simulink model "WESDem_SelectParam"  (R2016b)
settings: configuration reference "CodeGenConfigSet" (kept outside this file)
values from neighbouring files (symbols this model uses):
  WESDem_facFdbkHi_CUR = Calibration.Parameter    [init_WESDem_SelectParam.m]
  WESDem_facFdbkHi_CURX = Calibration.Parameter    [init_WESDem_SelectParam.m]
  WESDem_facFdbkHiParSet0_C = Calibration.Parameter    [init_WESDem_SelectParam.m]
  WESDem_facFdbkHiParSet1_C = Calibration.Parameter    [init_WESDem_SelectParam.m]
  WESDem_facFdbkHiParSet2_C = Calibration.Parameter    [init_WESDem_SelectParam.m]
  WESDem_facFdbkHiParSet3_C = Calibration.Parameter    [init_WESDem_SelectParam.m]
  WESDem_facFdbkLo_CUR = Calibration.Parameter    [init_WESDem_SelectParam.m]
  WESDem_facFdbkLo_CURX = Calibration.Parameter    [init_WESDem_SelectParam.m]
  WESDem_facFdbkLoParSet0_C = Calibration.Parameter    [init_WESDem_SelectParam.m]
  WESDem_facFdbkLoParSet1_C = Calibration.Parameter    [init_WESDem_SelectParam.m]
  WESDem_facFdbkLoParSet2_C = Calibration.Parameter    [init_WESDem_SelectParam.m]
  WESDem_facFdbkLoParSet3_C = Calibration.Parameter    [init_WESDem_SelectParam.m]
  WESDem_facFdbkMax_C = Calibration.Parameter    [init_WESDem_SelectParam.m]
  WESDem_facFdbkMin_C = Calibration.Parameter    [init_WESDem_SelectParam.m]
  WESDem_facFdbkTrqLosHiParSet0_C = Calibration.Parameter    [init_WESDem_SelectParam.m]
  WESDem_facFdbkTrqLosHiParSet1_C = Calibration.Parameter    [init_WESDem_SelectParam.m]
  WESDem_facFdbkTrqLosHiParSet2_C = Calibration.Parameter    [init_WESDem_SelectParam.m]
  WESDem_facFdbkTrqLosHiParSet3_C = Calibration.Parameter    [init_WESDem_SelectParam.m]
  WESDem_facFdbkTrqLosLoParSet0_C = Calibration.Parameter    [init_WESDem_SelectParam.m]
  WESDem_facFdbkTrqLosLoParSet1_C = Calibration.Parameter    [init_WESDem_SelectParam.m]
  WESDem_facFdbkTrqLosLoParSet2_C = Calibration.Parameter    [init_WESDem_SelectParam.m]
  WESDem_facFdbkTrqLosLoParSet3_C = Calibration.Parameter    [init_WESDem_SelectParam.m]
  WESDem_InrtVehParSet0_C = Calibration.Parameter    [init_WESDem_SelectParam.m]
  WESDem_InrtVehParSet1_C = Calibration.Parameter    [init_WESDem_SelectParam.m]
  WESDem_InrtVehParSet2_C = Calibration.Parameter    [init_WESDem_SelectParam.m]
  WESDem_InrtVehParSet3_C = Calibration.Parameter    [init_WESDem_SelectParam.m]
  WESDem_KiCorTempFac_MAP = Calibration.Parameter    [init_WESDem_SelectParam.m]
  WESDem_KiCorTempFac_MAPX = Calibration.Parameter    [init_WESDem_SelectParam.m]
  WESDem_KiCorTempFac_MAPY = Calibration.Parameter    [init_WESDem_SelectParam.m]
  WESDem_KiCorTrqFac_MAP = Calibration.Parameter    [init_WESDem_SelectParam.m]
  WESDem_KiCorTrqFac_MAPX = Calibration.Parameter    [init_WESDem_SelectParam.m]
  WESDem_KiCorTrqFac_MAPY = Calibration.Parameter    [init_WESDem_SelectParam.m]
  WESDem_KpCorTempFac_MAP = Calibration.Parameter    [init_WESDem_SelectParam.m]
  WESDem_KpCorTempFac_MAPX = Calibration.Parameter    [init_WESDem_SelectParam.m]
  WESDem_KpCorTempFac_MAPY = Calibration.Parameter    [init_WESDem_SelectParam.m]
  WESDem_KpCorTrqFac_MAP = Calibration.Parameter    [init_WESDem_SelectParam.m]
  WESDem_KpCorTrqFac_MAPX = Calibration.Parameter    [init_WESDem_SelectParam.m]
  WESDem_KpCorTrqFac_MAPY = Calibration.Parameter    [init_WESDem_SelectParam.m]
  WESDem_Par0dnAccLim_C = Calibration.Parameter    [init_WESDem_SelectParam.m]
  WESDem_Par0dnDeclLim_C = Calibration.Parameter    [init_WESDem_SelectParam.m]
  WESDem_Par0dnDeclLimBrk_C = Calibration.Parameter    [init_WESDem_SelectParam.m]
  WESDem_Par0EISGovCfg_C = Calibration.Parameter    [init_WESDem_SelectParam.m]
  WESDem_Par0IKi_C = Calibration.Parameter    [init_WESDem_SelectParam.m]
  WESDem_Par0IKiNeg_C = Calibration.Parameter    [init_WESDem_SelectParam.m]
  WESDem_Par0IKiPos_C = Calibration.Parameter    [init_WESDem_SelectParam.m]
  WESDem_Par0nIWinNeg_C = Calibration.Parameter    [init_WESDem_SelectParam.m]
  WESDem_Par0nIWinPos_C = Calibration.Parameter    [init_WESDem_SelectParam.m]
  WESDem_Par0nPWinNeg_C = Calibration.Parameter    [init_WESDem_SelectParam.m]
  WESDem_Par0nPWinPos_C = Calibration.Parameter    [init_WESDem_SelectParam.m]
  WESDem_Par0PKp_C = Calibration.Parameter    [init_WESDem_SelectParam.m]
  WESDem_Par0PKpNeg_C = Calibration.Parameter    [init_WESDem_SelectParam.m]
  WESDem_Par0PKpPos_C = Calibration.Parameter    [init_WESDem_SelectParam.m]
  WESDem_Par1dnAccLim_C = Calibration.Parameter    [init_WESDem_SelectParam.m]
  WESDem_Par1dnDeclLim_C = Calibration.Parameter    [init_WESDem_SelectParam.m]
  WESDem_Par1dnDeclLimBrk_C = Calibration.Parameter    [init_WESDem_SelectParam.m]
  WESDem_Par1EISGovCfg_C = Calibration.Parameter    [init_WESDem_SelectParam.m]
  WESDem_Par1IKi_C = Calibration.Parameter    [init_WESDem_SelectParam.m]
  WESDem_Par1IKiNeg_C = Calibration.Parameter    [init_WESDem_SelectParam.m]
  WESDem_Par1IKiPos_C = Calibration.Parameter    [init_WESDem_SelectParam.m]
  WESDem_Par1nIWinNeg_C = Calibration.Parameter    [init_WESDem_SelectParam.m]
  WESDem_Par1nIWinPos_C = Calibration.Parameter    [init_WESDem_SelectParam.m]
  WESDem_Par1nPWinNeg_C = Calibration.Parameter    [init_WESDem_SelectParam.m]
  WESDem_Par1nPWinPos_C = Calibration.Parameter    [init_WESDem_SelectParam.m]
  WESDem_Par1PKp_C = Calibration.Parameter    [init_WESDem_SelectParam.m]
  WESDem_Par1PKpNeg_C = Calibration.Parameter    [init_WESDem_SelectParam.m]
  WESDem_Par1PKpPos_C = Calibration.Parameter    [init_WESDem_SelectParam.m]
  WESDem_Par2dnAccLim_C = Calibration.Parameter    [init_WESDem_SelectParam.m]
  WESDem_Par2dnDeclLim_C = Calibration.Parameter    [init_WESDem_SelectParam.m]
  WESDem_Par2dnDeclLimBrk_C = Calibration.Parameter    [init_WESDem_SelectParam.m]
  WESDem_Par2EISGovCfg_C = Calibration.Parameter    [init_WESDem_SelectParam.m]
  WESDem_Par2IKi_C = Calibration.Parameter    [init_WESDem_SelectParam.m]
  WESDem_Par2IKiNeg_C = Calibration.Parameter    [init_WESDem_SelectParam.m]
  WESDem_Par2IKiPos_C = Calibration.Parameter    [init_WESDem_SelectParam.m]
  WESDem_Par2nIWinNeg_C = Calibration.Parameter    [init_WESDem_SelectParam.m]
  WESDem_Par2nIWinPos_C = Calibration.Parameter    [init_WESDem_SelectParam.m]
  WESDem_Par2nPWinNeg_C = Calibration.Parameter    [init_WESDem_SelectParam.m]
  WESDem_Par2nPWinPos_C = Calibration.Parameter    [init_WESDem_SelectParam.m]
  WESDem_Par2PKp_C = Calibration.Parameter    [init_WESDem_SelectParam.m]
  WESDem_Par2PKpNeg_C = Calibration.Parameter    [init_WESDem_SelectParam.m]
  WESDem_Par2PKpPos_C = Calibration.Parameter    [init_WESDem_SelectParam.m]
  WESDem_Par3dnAccLim_C = Calibration.Parameter    [init_WESDem_SelectParam.m]
  WESDem_Par3dnDeclLim_C = Calibration.Parameter    [init_WESDem_SelectParam.m]
  WESDem_Par3dnDeclLimBrk_C = Calibration.Parameter    [init_WESDem_SelectParam.m]
  WESDem_Par3EISGovCfg_C = Calibration.Parameter    [init_WESDem_SelectParam.m]
  WESDem_Par3IKi_C = Calibration.Parameter    [init_WESDem_SelectParam.m]
  WESDem_Par3IKiNeg_C = Calibration.Parameter    [init_WESDem_SelectParam.m]
  WESDem_Par3IKiPos_C = Calibration.Parameter    [init_WESDem_SelectParam.m]
  WESDem_Par3nIWinNeg_C = Calibration.Parameter    [init_WESDem_SelectParam.m]
  WESDem_Par3nIWinPos_C = Calibration.Parameter    [init_WESDem_SelectParam.m]
  WESDem_Par3nPWinNeg_C = Calibration.Parameter    [init_WESDem_SelectParam.m]
  WESDem_Par3nPWinPos_C = Calibration.Parameter    [init_WESDem_SelectParam.m]
  WESDem_Par3PKp_C = Calibration.Parameter    [init_WESDem_SelectParam.m]
  WESDem_Par3PKpNeg_C = Calibration.Parameter    [init_WESDem_SelectParam.m]
  WESDem_Par3PKpPos_C = Calibration.Parameter    [init_WESDem_SelectParam.m]
  WESDem_swtFacFdbkSelHi_C = Calibration.Parameter    [init_WESDem_SelectParam.m]
  WESDem_swtFacFdbkSelLo_C = Calibration.Parameter    [init_WESDem_SelectParam.m]
  WESDem_swtNSelCorFac_C = Calibration.Parameter    [init_WESDem_SelectParam.m]
  WESDem_swtParCorActv_C = Calibration.Parameter    [init_WESDem_SelectParam.m]
  WESDem_swtTempSel_C = Calibration.Parameter    [init_WESDem_SelectParam.m]
  WESDem_swtTrqSelCorFac_C = Calibration.Parameter    [init_WESDem_SelectParam.m]
  WESDem_tiFltTrqLosParSet0_C = Calibration.Parameter    [init_WESDem_SelectParam.m]
  WESDem_tiFltTrqLosParSet1_C = Calibration.Parameter    [init_WESDem_SelectParam.m]
  WESDem_tiFltTrqLosParSet2_C = Calibration.Parameter    [init_WESDem_SelectParam.m]
  WESDem_tiFltTrqLosParSet3_C = Calibration.Parameter    [init_WESDem_SelectParam.m]
  WESDem_tiNAvrgPT1CorFac_C = Calibration.Parameter    [init_WESDem_SelectParam.m]
  WESDem_tiTrqPT1CorFac_C = Calibration.Parameter    [init_WESDem_SelectParam.m]
undefined symbols (not defined in the file or in its folder): Switch_conv
libraries: CXLib x6
settings Model: Creator=zhoukai  LastModifiedBy=zhoukai
settings ConfigSetRef: SourceLocation=Base Workspace

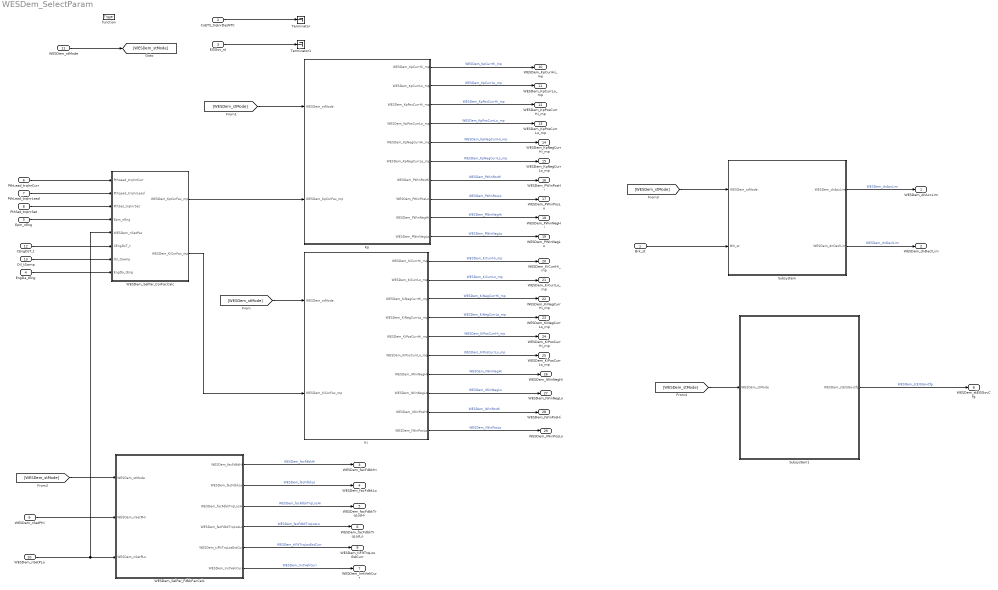
== system WESDem_SelectParam ==
  Brk_st : Inport  Description=Brake switch state  OutMin=0  OutMax=255  OutDataTypeStr=State_uint8
  CoETS_trqInrDesNTC : Inport  Tag=Nm  Description=Additional desired engine friction Nm  Port=2  OutMin=-3276  OutMax=3276  OutDataTypeStr=Trq_Nm
  EISGov_st : Inport  Description=Status information of EISGov and its clients  Port=3  OutMin=0  OutMax=2147483648  OutDataTypeStr=State_uint32
  EngDa_tEng : Inport  Tag=deg  Description=Engine temperature  Port=4  OutMin=-1000  OutMax=1000  OutDataTypeStr=Temp_deg
  Epm_nEng : Inport  Tag=rpm  Description=Engine speed  Port=5  OutMin=0  OutMax=6000  OutDataTypeStr=EngSpeed_rpm
  PthLead_trqInrCurr : Inport  Tag=Nm  Description=Actual percent engine torque  Port=6  OutMin=-3000  OutMax=3000  OutDataTypeStr=Trq_Nm
  PthLead_trqInrLead : Inport  Tag=Nm  Description=Inner torque lead value  Port=7  OutMin=-3000  OutMax=3000  OutDataTypeStr=Trq_Nm
  PthSet_trqInrSet : Inport  Tag=Nm  Description=Inner torque set value after monitoring limitation  Port=8  OutMin=-3000  OutMax=3276.7  OutDataTypeStr=Trq_Nm
  WESDem_nSetPHi : Inport  Tag=rpm  Description=Higher setpoint speed interval of WESDem  Port=9  OutMin=0  OutMax=6000  OutDataTypeStr=EngSpeed_rpm
  WESDem_nSetPLo : Inport  Tag=rpm  Description=Lower setpoint speed interval of WESDem  Port=10  OutMin=0  OutMax=6000  OutDataTypeStr=EngSpeed_rpm
  WESDem_stMode : Inport  Description=Operating mode of the working engine speed demand  Port=11  OutMin=0  OutMax=255  OutDataTypeStr=State_uint8
  CEngDsT_t : Inport  Tag=deg  Description=engine coolant temperature after filter  Port=12  OutMin=-200  OutMax=200  OutDataTypeStr=Temp_deg
  Oil_tSwmp : Inport  Tag=deg  Description=Oil temperature in oil sump  Port=13  OutMin=-50  OutMax=200  OutDataTypeStr=Temp_deg
  function : TriggerPort  TriggerType=function-call  VariantControl=Variant
  "Ki " : Subsystem
  "Kp " : Subsystem
  Subsystem : Subsystem
  Subsystem1 : Subsystem
  Terminator : Terminator
  Terminator1 : Terminator
  WESDem_SelPar_CorFacCalc : Subsystem
  WESDem_SelPar_FdbkFacCalc : Subsystem
  WESDem_dnAccLim : Outport  Tag=rpm/s  Description=Maximum permissible acceleration (Engine speed)  OutMin=-12000  OutMax=12000  OutDataTypeStr=EngSpeed_rpm_s
  WESDem_dnDeclLim : Outport  Tag=rpm/s  Description=Maximum permissible deceleration (Engine speed)  Port=2  OutMin=-12000  OutMax=12000  OutDataTypeStr=EngSpeed_rpm_s
  WESDem_facFdbkHi : Outport  Tag=rpm/Nm  Description=Feedback factor for the higher setpoint  Port=3  OutMin=-20  OutMax=20  OutDataTypeStr=FdbkNm2rpm_rpm_Nm
  WESDem_facFdbkLo : Outport  Tag=rpm/Nm  Description=Feedback factor for the lower setpoint  Port=4  OutMin=-20  OutMax=20  OutDataTypeStr=FdbkNm2rpm_rpm_Nm
  WESDem_facFdbkTrqLosHi : Outport  Tag=rpm/Nm  Description=inner feedback factor for the upper setpoint  Port=5  OutMin=-20  OutMax=20  OutDataTypeStr=FdbkNm2rpm_rpm_Nm
  WESDem_facFdbkTrqLosLo : Outport  Tag=rpm/Nm  Description=inner feedback factor for the lower setpoint  Port=6  OutMin=-20  OutMax=20  OutDataTypeStr=FdbkNm2rpm_rpm_Nm
  WESDem_InrtVehCurr : Outport  Tag=Nm/(rpm/s)  Description=mass inertia for EISGov torque loss estimation  Port=7  OutMin=-50  OutMax=50  OutDataTypeStr=HLSDem_Inrt
  WESDem_stEISGovCfg : Outport  Description=Configuration of the EISGov  Port=8  OutMin=0  OutMax=255  OutDataTypeStr=State_uint8
  WESDem_tiFltTrqLosEstCurr : Outport  Description=time constant (PT1-Filter) for EISGov torque loss estimation  Port=9  OutMin=0  OutMax=99.998  OutDataTypeStr=PT_fac
  WESDem_KpCurrHi_mp : Outport  Tag=Nm/rpm  Description=Current small signal gain for the higher P component  Port=10  OutMin=-10000  OutMax=10000  OutDataTypeStr=HLSDem_Kp
  WESDem_KpCurrLo_mp : Outport  Tag=Nm/rpm  Description=Current small signal gain for the lower P component  Port=11  OutMin=-10000  OutMax=10000  OutDataTypeStr=HLSDem_Kp
  WESDem_KpPosCurrHi_mp : Outport  Tag=Nm/rpm  Description=Current positive large signal gain for the higher P component  Port=12  OutMin=-10000  OutMax=10000  OutDataTypeStr=HLSDem_Kp
  WESDem_KpPosCurrLo_mp : Outport  Tag=Nm/rpm  Description=Current positive large signal gain for the lower P component  Port=13  OutMin=-10000  OutMax=10000  OutDataTypeStr=HLSDem_Kp
  WESDem_KpNegCurrHi_mp : Outport  Tag=Nm/rpm  Description=Current negative large signal gain for the higher P component  Port=14  OutMin=-10000  OutMax=10000  OutDataTypeStr=HLSDem_Kp
  WESDem_KpNegCurrLo_mp : Outport  Tag=Nm/rpm  Description=Current negative large signal gain for the lower P component  Port=15  OutMin=-10000  OutMax=10000  OutDataTypeStr=HLSDem_Kp
  WESDem_PWinPosHi : Outport  Tag=rpm  Description=Positive higher small signal window for proportional component  Port=16  OutMin=-6000  OutMax=6000  OutDataTypeStr=EngSpeed_rpm
  WESDem_PWinPosLo : Outport  Tag=rpm  Description=Positive lower small signal window for proportional component  Port=17  OutMin=-6000  OutMax=6000  OutDataTypeStr=EngSpeed_rpm
  WESDem_PWinNegHi : Outport  Tag=rpm  Description=Negative higher small signal window for proportional component  Port=18  OutMin=-6000  OutMax=6000  OutDataTypeStr=EngSpeed_rpm
  WESDem_PWinNegLo : Outport  Tag=rpm  Description=Negative lower small signal window for proportional component  Port=19  OutMin=-6000  OutMax=6000  OutDataTypeStr=EngSpeed_rpm
  WESDem_KiCurrHi_mp : Outport  Tag=Nm/(rpm*s)  Description=Current small signal gain for the higher I component  Port=20  OutMin=-18000  OutMax=18000  OutDataTypeStr=HLSDem_Ki
  WESDem_KiCurrLo_mp : Outport  Tag=Nm/(rpm*s)  Description=Current small signal gain for the lower I component  Port=21  OutMin=-18000  OutMax=18000  OutDataTypeStr=HLSDem_Ki
  WESDem_KiNegCurrHi_mp : Outport  Tag=Nm/(rpm*s)  Description=Current negative large signal gain for the higher I component  Port=22  OutMin=-18000  OutMax=18000  OutDataTypeStr=HLSDem_Ki
  WESDem_KiNegCurrLo_mp : Outport  Tag=Nm/(rpm*s)  Description=Current negative large signal gain for the lower I component  Port=23  OutMin=-18000  OutMax=18000  OutDataTypeStr=HLSDem_Ki
  WESDem_KiPosCurrHi_mp : Outport  Tag=Nm/(rpm*s)  Description=Current positive large signal gain for the higher I component  Port=24  OutMin=-18000  OutMax=18000  OutDataTypeStr=HLSDem_Ki
  WESDem_KiPosCurrLo_mp : Outport  Tag=Nm/(rpm*s)  Description=Current positive large signal gain for the lower I component  Port=25  OutMin=-18000  OutMax=18000  OutDataTypeStr=HLSDem_Ki
  WESDem_IWinNegHi : Outport  Tag=rpm  Description=Negative higher small signal window for integral component  Port=26  OutMin=-6000  OutMax=6000  OutDataTypeStr=EngSpeed_rpm
  WESDem_IWinNegLo : Outport  Tag=rpm  Description=Negative lower small signal window for integral component  Port=27  OutMin=-6000  OutMax=6000  OutDataTypeStr=EngSpeed_rpm
  WESDem_IWinPosHi : Outport  Tag=rpm  Description=Positive higher small signal window for integral component  Port=28  OutMin=-6000  OutMax=6000  OutDataTypeStr=EngSpeed_rpm
  WESDem_IWinPosLo : Outport  Tag=rpm  Description=Positive lower small signal window for integral component  Port=29  OutMin=-6000  OutMax=6000  OutDataTypeStr=EngSpeed_rpm
  wires:
  WESDem_SelPar_CorFacCalc/2(WESDem_KiCorFac_mp) -> "Ki "/2(WESDem_KiCorFac_mp)
  WESDem_SelPar_CorFacCalc/1(WESDem_KpCorFac_mp) -> "Kp "/2(WESDem_KpCorFac_mp)
  WESDem_stMode/1 -> [WESDem_stMode]
  [WESDem_stMode] -> "Ki "/1(WESDem_stMode)
  [WESDem_stMode] -> "Kp "/1(WESDem_stMode)
  PthLead_trqInrCurr/1 -> WESDem_SelPar_CorFacCalc/1(PthLead_trqInrCurr)
  PthLead_trqInrLead/1 -> WESDem_SelPar_CorFacCalc/2(PthLead_trqInrLead)
  PthSet_trqInrSet/1 -> WESDem_SelPar_CorFacCalc/3(PthSet_trqInrSet)
  Epm_nEng/1 -> WESDem_SelPar_CorFacCalc/4(Epm_nEng)
  EngDa_tEng/1 -> WESDem_SelPar_CorFacCalc/8(EngDa_tEng)
  CEngDsT_t/1 -> WESDem_SelPar_CorFacCalc/6(CEngDsT_t)
  Oil_tSwmp/1 -> WESDem_SelPar_CorFacCalc/7(Oil_tSwmp)
  WESDem_nSetPHi/1 -> WESDem_SelPar_FdbkFacCalc/2(WESDem_nSetPHi)
  WESDem_nSetPLo/1 -> WESDem_SelPar_CorFacCalc/5(WESDem_nSetPLo), WESDem_SelPar_FdbkFacCalc/3(WESDem_nSetPLo)
  [WESDem_stMode] -> WESDem_SelPar_FdbkFacCalc/1(WESDem_stMode)
  Brk_st/1 -> Subsystem/2(Brk_st)
  [WESDem_stMode] -> Subsystem/1(WESDem_stMode)
  [WESDem_stMode] -> Subsystem1/1(WESDem_stMode)
  Subsystem/2(WESDem_dnDeclLim) -> WESDem_dnDeclLim/1  "WESDem_dnDeclLim"
  Subsystem/1(WESDem_dnAccLim) -> WESDem_dnAccLim/1  "WESDem_dnAccLim"
  Subsystem1/1(WESDem_stEISGovCfg) -> WESDem_stEISGovCfg/1  "WESDem_stEISGovCfg"
  WESDem_SelPar_FdbkFacCalc/1(WESDem_facFdbkHi) -> WESDem_facFdbkHi/1  "WESDem_facFdbkHi"
  WESDem_SelPar_FdbkFacCalc/2(WESDem_facFdbkLo) -> WESDem_facFdbkLo/1  "WESDem_facFdbkLo"
  WESDem_SelPar_FdbkFacCalc/3(WESDem_facFdbkTrqLosHi) -> WESDem_facFdbkTrqLosHi/1  "WESDem_facFdbkTrqLosHi"
  WESDem_SelPar_FdbkFacCalc/4(WESDem_facFdbkTrqLosLo) -> WESDem_facFdbkTrqLosLo/1  "WESDem_facFdbkTrqLosLo"
  WESDem_SelPar_FdbkFacCalc/6(WESDem_InrtVehCurr) -> WESDem_InrtVehCurr/1  "WESDem_InrtVehCurr"
  WESDem_SelPar_FdbkFacCalc/5(WESDem_tiFltTrqLosEstCurr) -> WESDem_tiFltTrqLosEstCurr/1  "WESDem_tiFltTrqLosEstCurr"
  CoETS_trqInrDesNTC/1 -> Terminator/1
  EISGov_st/1 -> Terminator1/1
  "Kp "/1(WESDem_KpCurrHi_mp) -> WESDem_KpCurrHi_mp/1  "WESDem_KpCurrHi_mp"
  "Kp "/2(WESDem_KpCurrLo_mp) -> WESDem_KpCurrLo_mp/1  "WESDem_KpCurrLo_mp"
  "Kp "/3(WESDem_KpPosCurrHi_mp) -> WESDem_KpPosCurrHi_mp/1  "WESDem_KpPosCurrHi_mp"
  "Kp "/4(WESDem_KpPosCurrLo_mp) -> WESDem_KpPosCurrLo_mp/1  "WESDem_KpPosCurrLo_mp"
  "Kp "/5(WESDem_KpNegCurrHi_mp) -> WESDem_KpNegCurrHi_mp/1  "WESDem_KpNegCurrHi_mp"
  "Kp "/6(WESDem_KpNegCurrLo_mp) -> WESDem_KpNegCurrLo_mp/1  "WESDem_KpNegCurrLo_mp"
  "Kp "/7(WESDem_PWinPosHi) -> WESDem_PWinPosHi/1  "WESDem_PWinPosHi"
  "Kp "/8(WESDem_PWinPosLo) -> WESDem_PWinPosLo/1  "WESDem_PWinPosLo"
  "Kp "/9(WESDem_PWinNegHi) -> WESDem_PWinNegHi/1  "WESDem_PWinNegHi"
  "Kp "/10(WESDem_PWinNegLo) -> WESDem_PWinNegLo/1  "WESDem_PWinNegLo"
  "Ki "/2(WESDem_KiCurrLo_mp) -> WESDem_KiCurrLo_mp/1  "WESDem_KiCurrLo_mp"
  "Ki "/3(WESDem_KiNegCurrHi_mp) -> WESDem_KiNegCurrHi_mp/1  "WESDem_KiNegCurrHi_mp"
  "Ki "/5(WESDem_KiPosCurrHi_mp) -> WESDem_KiPosCurrHi_mp/1  "WESDem_KiPosCurrHi_mp"
  "Ki "/6(WESDem_KiPosCurrLo_mp) -> WESDem_KiPosCurrLo_mp/1  "WESDem_KiPosCurrLo_mp"
  "Ki "/7(WESDem_IWinNegHi) -> WESDem_IWinNegHi/1  "WESDem_IWinNegHi"
  "Ki "/8(WESDem_IWinNegLo) -> WESDem_IWinNegLo/1  "WESDem_IWinNegLo"
  "Ki "/9(WESDem_IWinPosHi) -> WESDem_IWinPosHi/1  "WESDem_IWinPosHi"
  "Ki "/10(WESDem_IWinPosLo) -> WESDem_IWinPosLo/1  "WESDem_IWinPosLo"
  "Ki "/4(WESDem_KiNegCurrLo_mp) -> WESDem_KiNegCurrLo_mp/1  "WESDem_KiNegCurrLo_mp"
  "Ki "/1(WESDem_KiCurrHi_mp) -> WESDem_KiCurrHi_mp/1  "WESDem_KiCurrHi_mp"

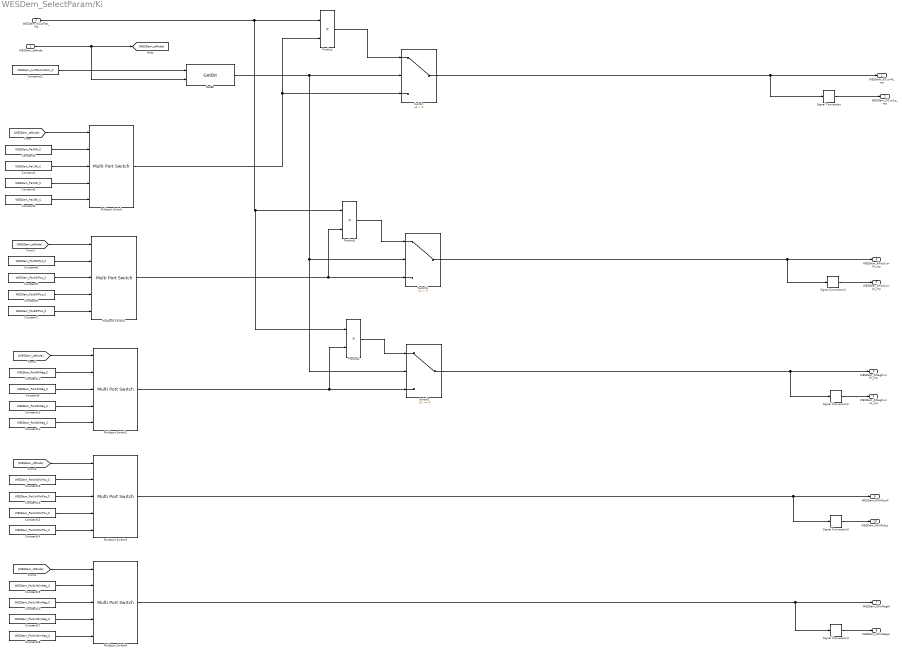
== system WESDem_SelectParam/Ki  ==
  WESDem_stMode : Inport  Description=Operating mode of the working engine speed demand  OutMin=0  OutMax=255  OutDataTypeStr=State_uint8
  WESDem_KiCorFac_mp : Inport  Port=2  OutDataTypeStr=Factor
  Constant1 : Constant  Value=WESDem_Par1IKi_C
  Constant10 : Constant  Value=WESDem_Par2IKiNeg_C
  Constant11 : Constant  Value=WESDem_Par3IKiNeg_C
  Constant12 : Constant  Value=WESDem_Par0IKiNeg_C
  Constant13 : Constant  Value=WESDem_Par2nIWinPos_C
  Constant14 : Constant  Value=WESDem_Par3nIWinPos_C
  Constant15 : Constant  Value=WESDem_Par0nIWinPos_C
  Constant16 : Constant  Value=WESDem_Par1nIWinPos_C
  Constant17 : Constant  Value=WESDem_Par2nIWinNeg_C
  Constant18 : Constant  Value=WESDem_Par3nIWinNeg_C
  Constant19 : Constant  Value=WESDem_Par0nIWinNeg_C
  Constant2 : Constant  Value=WESDem_Par2IKi_C
  Constant20 : Constant  Value=WESDem_Par1nIWinNeg_C
  Constant21 : Constant  Value=WESDem_swtParCorActv_C
  Constant3 : Constant  Value=WESDem_Par3IKi_C
  Constant4 : Constant  Value=WESDem_Par0IKi_C
  Constant5 : Constant  Value=WESDem_Par1IKiPos_C
  Constant6 : Constant  Value=WESDem_Par2IKiPos_C
  Constant7 : Constant  Value=WESDem_Par3IKiPos_C
  Constant8 : Constant  Value=WESDem_Par0IKiPos_C
  Constant9 : Constant  Value=WESDem_Par1IKiNeg_C
  GetBit : CXLib/GetBit  dataTypeString=uint8  dataLength=0
      settings: AttributesFormatString=Get bit from %<dataTypeString>
  Multiport Switch{,1..4} (5 alike) : MultiPortSwitch  DataPortOrder=Zero-based contiguous  Inputs=4
  Product : Product  OutDataTypeStr=Inherit: Inherit via back propagation  SaturateOnIntegerOverflow=on
  Product1 : Product  OutDataTypeStr=Inherit: Inherit via back propagation  SaturateOnIntegerOverflow=on
  Product2 : Product  OutDataTypeStr=Inherit: Inherit via back propagation  SaturateOnIntegerOverflow=on
  Signal Conversion{,1..4} (5 alike) : SignalConversion  OverrideOpt=off
  Switch : Switch  Criteria=u2 > Threshold  OutDataTypeStr=Inherit: Inherit via back propagation
  Switch1 : Switch  Criteria=u2 > Threshold
  Switch2 : Switch  Criteria=u2 ~= 0
  WESDem_KiCurrHi_mp : Outport  Tag=Nm/(rpm*s)  Description=Current small signal gain for the higher I component  OutMin=-18000  OutMax=18000  OutDataTypeStr=HLSDem_Ki
  WESDem_KiCurrLo_mp : Outport  Tag=Nm/(rpm*s)  Description=Current small signal gain for the lower I component  Port=2  OutMin=-18000  OutMax=18000  OutDataTypeStr=HLSDem_Ki
  WESDem_KiNegCurrHi_mp : Outport  Tag=Nm/(rpm*s)  Description=Current negative large signal gain for the higher I component  Port=3  OutMin=-18000  OutMax=18000  OutDataTypeStr=HLSDem_Ki
  WESDem_KiNegCurrLo_mp : Outport  Tag=Nm/(rpm*s)  Description=Current negative large signal gain for the lower I component  Port=4  OutMin=-18000  OutMax=18000  OutDataTypeStr=HLSDem_Ki
  WESDem_KiPosCurrHi_mp : Outport  Tag=Nm/(rpm*s)  Description=Current positive large signal gain for the higher I component  Port=5  OutMin=-18000  OutMax=18000  OutDataTypeStr=HLSDem_Ki
  WESDem_KiPosCurrLo_mp : Outport  Tag=Nm/(rpm*s)  Description=Current positive large signal gain for the lower I component  Port=6  OutMin=-18000  OutMax=18000  OutDataTypeStr=HLSDem_Ki
  WESDem_IWinNegHi : Outport  Tag=rpm  Description=Negative higher small signal window for integral component  Port=7  OutMin=-6000  OutMax=6000  OutDataTypeStr=EngSpeed_rpm
  WESDem_IWinNegLo : Outport  Tag=rpm  Description=Negative lower small signal window for integral component  Port=8  OutMin=-6000  OutMax=6000  OutDataTypeStr=EngSpeed_rpm
  WESDem_IWinPosHi : Outport  Tag=rpm  Description=Positive higher small signal window for integral component  Port=9  OutMin=-6000  OutMax=6000  OutDataTypeStr=EngSpeed_rpm
  WESDem_IWinPosLo : Outport  Tag=rpm  Description=Positive lower small signal window for integral component  Port=10  OutMin=-6000  OutMax=6000  OutDataTypeStr=EngSpeed_rpm
  wires:
  WESDem_stMode/1 -> GetBit/2, [WESDem_stMode]
  [WESDem_stMode] -> Multiport Switch/1
  Constant4/1 -> Multiport Switch/2
  Constant1/1 -> Multiport Switch/3
  Constant2/1 -> Multiport Switch/4
  Constant3/1 -> Multiport Switch/5
  [WESDem_stMode] -> Multiport Switch1/1
  Constant8/1 -> Multiport Switch1/2
  Constant5/1 -> Multiport Switch1/3
  Constant6/1 -> Multiport Switch1/4
  Constant7/1 -> Multiport Switch1/5
  [WESDem_stMode] -> Multiport Switch2/1
  Constant12/1 -> Multiport Switch2/2
  Constant9/1 -> Multiport Switch2/3
  Constant10/1 -> Multiport Switch2/4
  Constant11/1 -> Multiport Switch2/5
  [WESDem_stMode] -> Multiport Switch3/1
  Constant15/1 -> Multiport Switch3/2
  Constant16/1 -> Multiport Switch3/3
  Constant13/1 -> Multiport Switch3/4
  Constant14/1 -> Multiport Switch3/5
  [WESDem_stMode] -> Multiport Switch4/1
  Constant19/1 -> Multiport Switch4/2
  Constant20/1 -> Multiport Switch4/3
  Constant17/1 -> Multiport Switch4/4
  Constant18/1 -> Multiport Switch4/5
  Constant21/1 -> GetBit/1
  GetBit/1 -> Switch2/2, Switch1/2, Switch/2
  Multiport Switch/1 -> Product/2, Switch/3
  Multiport Switch1/1 -> Product1/2, Switch1/3
  WESDem_KiCorFac_mp/1 -> Product2/1, Product1/1, Product/1
  Product/1 -> Switch/1
  Product1/1 -> Switch1/1
  Multiport Switch2/1 -> Product2/2, Switch2/3
  Product2/1 -> Switch2/1
  Switch/1 -> Signal Conversion/1, WESDem_KiCurrHi_mp/1
  Switch1/1 -> Signal Conversion1/1, WESDem_KiPosCurrHi_mp/1
  Switch2/1 -> Signal Conversion2/1, WESDem_KiNegCurrHi_mp/1
  Multiport Switch3/1 -> Signal Conversion3/1, WESDem_IWinPosHi/1
  Multiport Switch4/1 -> Signal Conversion4/1, WESDem_IWinNegHi/1
  Signal Conversion/1 -> WESDem_KiCurrLo_mp/1
  Signal Conversion1/1 -> WESDem_KiPosCurrLo_mp/1
  Signal Conversion2/1 -> WESDem_KiNegCurrLo_mp/1
  Signal Conversion3/1 -> WESDem_IWinPosLo/1
  Signal Conversion4/1 -> WESDem_IWinNegLo/1

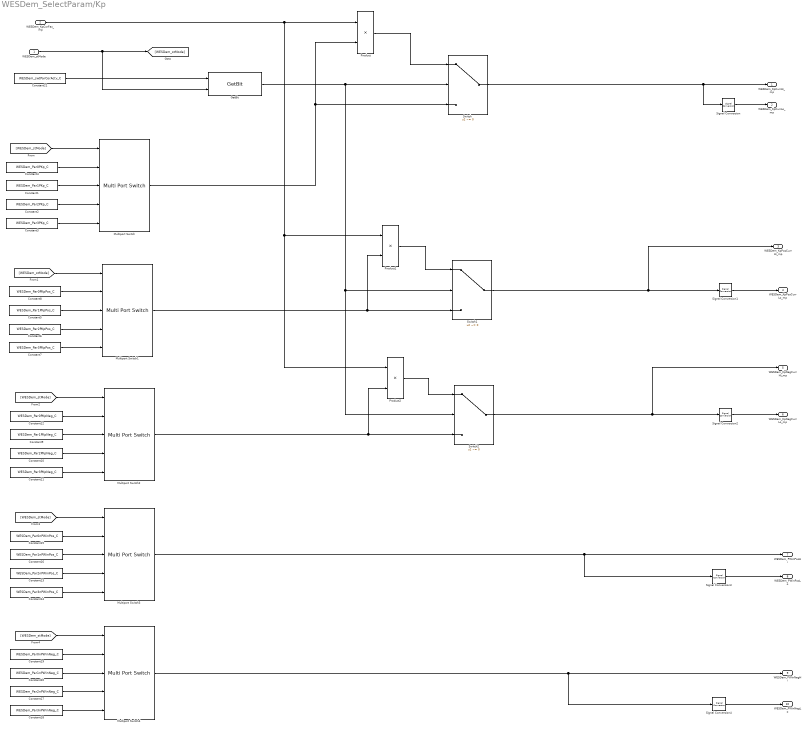
== system WESDem_SelectParam/Kp  ==
  WESDem_stMode : Inport  Description=Operating mode of the working engine speed demand  OutMin=0  OutMax=255  OutDataTypeStr=State_uint8
  WESDem_KpCorFac_mp : Inport  Port=2  OutDataTypeStr=Factor
  Constant1 : Constant  Value=WESDem_Par1PKp_C
  Constant10 : Constant  Value=WESDem_Par2PKpNeg_C
  Constant11 : Constant  Value=WESDem_Par3PKpNeg_C
  Constant12 : Constant  Value=WESDem_Par0PKpNeg_C
  Constant13 : Constant  Value=WESDem_Par2nPWinPos_C
  Constant14 : Constant  Value=WESDem_Par3nPWinPos_C
  Constant15 : Constant  Value=WESDem_Par0nPWinPos_C
  Constant16 : Constant  Value=WESDem_Par1nPWinPos_C
  Constant17 : Constant  Value=WESDem_Par2nPWinNeg_C
  Constant18 : Constant  Value=WESDem_Par3nPWinNeg_C
  Constant19 : Constant  Value=WESDem_Par0nPWinNeg_C
  Constant2 : Constant  Value=WESDem_Par2PKp_C
  Constant20 : Constant  Value=WESDem_Par1nPWinNeg_C
  Constant21 : Constant  Value=WESDem_swtParCorActv_C
  Constant3 : Constant  Value=WESDem_Par3PKp_C
  Constant4 : Constant  Value=WESDem_Par0PKp_C
  Constant5 : Constant  Value=WESDem_Par1PKpPos_C
  Constant6 : Constant  Value=WESDem_Par2PKpPos_C
  Constant7 : Constant  Value=WESDem_Par3PKpPos_C
  Constant8 : Constant  Value=WESDem_Par0PKpPos_C
  Constant9 : Constant  Value=WESDem_Par1PKpNeg_C
  GetBit : CXLib/GetBit  dataTypeString=uint8  dataLength=0
      settings: AttributesFormatString=Get bit from %<dataTypeString>
  Multiport Switch{,1..4} (5 alike) : MultiPortSwitch  DataPortOrder=Zero-based contiguous  Inputs=4
  Product : Product  OutDataTypeStr=Inherit: Inherit via back propagation  SaturateOnIntegerOverflow=on
  Product1 : Product  OutDataTypeStr=Inherit: Inherit via back propagation  SaturateOnIntegerOverflow=on
  Product2 : Product  OutDataTypeStr=Inherit: Inherit via back propagation  SaturateOnIntegerOverflow=on
  Signal Conversion{,1..4} (5 alike) : SignalConversion  OverrideOpt=off
  Switch : Switch  Criteria=u2 ~= 0
  Switch1 : Switch  Criteria=u2 ~= 0  OutDataTypeStr=Inherit: Inherit via back propagation
  Switch2 : Switch  Criteria=u2 ~= 0  OutDataTypeStr=Inherit: Inherit via back propagation
  WESDem_KpCurrHi_mp : Outport  Tag=Nm/rpm  Description=Current small signal gain for the higher P component  OutMin=-10000  OutMax=10000  OutDataTypeStr=HLSDem_Kp
  WESDem_KpCurrLo_mp : Outport  Tag=Nm/rpm  Description=Current small signal gain for the lower P component  Port=2  OutMin=-10000  OutMax=10000  OutDataTypeStr=HLSDem_Kp
  WESDem_KpPosCurrHi_mp : Outport  Tag=Nm/rpm  Description=Current positive large signal gain for the higher P component  Port=3  OutMin=-10000  OutMax=10000  OutDataTypeStr=HLSDem_Kp
  WESDem_KpPosCurrLo_mp : Outport  Tag=Nm/rpm  Description=Current positive large signal gain for the lower P component  Port=4  OutMin=-10000  OutMax=10000  OutDataTypeStr=HLSDem_Kp
  WESDem_KpNegCurrHi_mp : Outport  Tag=Nm/rpm  Description=Current negative large signal gain for the higher P component  Port=5  OutMin=-10000  OutMax=10000  OutDataTypeStr=HLSDem_Kp
  WESDem_KpNegCurrLo_mp : Outport  Tag=Nm/rpm  Description=Current negative large signal gain for the lower P component  Port=6  OutMin=-10000  OutMax=10000  OutDataTypeStr=HLSDem_Kp
  WESDem_PWinPosHi : Outport  Tag=rpm  Description=Positive higher small signal window for proportional component  Port=7  OutMin=-6000  OutMax=6000  OutDataTypeStr=EngSpeed_rpm
  WESDem_PWinPosLo : Outport  Tag=rpm  Description=Positive lower small signal window for proportional component  Port=8  OutMin=-6000  OutMax=6000  OutDataTypeStr=EngSpeed_rpm
  WESDem_PWinNegHi : Outport  Tag=rpm  Description=Negative higher small signal window for proportional component  Port=9  OutMin=-6000  OutMax=6000  OutDataTypeStr=EngSpeed_rpm
  WESDem_PWinNegLo : Outport  Tag=rpm  Description=Negative lower small signal window for proportional component  Port=10  OutMin=-6000  OutMax=6000  OutDataTypeStr=EngSpeed_rpm
  wires:
  WESDem_stMode/1 -> GetBit/2, [WESDem_stMode]
  [WESDem_stMode] -> Multiport Switch/1
  Constant4/1 -> Multiport Switch/2
  Constant1/1 -> Multiport Switch/3
  Constant2/1 -> Multiport Switch/4
  Constant3/1 -> Multiport Switch/5
  [WESDem_stMode] -> Multiport Switch1/1
  Constant8/1 -> Multiport Switch1/2
  Constant5/1 -> Multiport Switch1/3
  Constant6/1 -> Multiport Switch1/4
  Constant7/1 -> Multiport Switch1/5
  [WESDem_stMode] -> Multiport Switch2/1
  Constant12/1 -> Multiport Switch2/2
  Constant9/1 -> Multiport Switch2/3
  Constant10/1 -> Multiport Switch2/4
  Constant11/1 -> Multiport Switch2/5
  [WESDem_stMode] -> Multiport Switch3/1
  Constant15/1 -> Multiport Switch3/2
  Constant16/1 -> Multiport Switch3/3
  Constant13/1 -> Multiport Switch3/4
  Constant14/1 -> Multiport Switch3/5
  [WESDem_stMode] -> Multiport Switch4/1
  Constant19/1 -> Multiport Switch4/2
  Constant20/1 -> Multiport Switch4/3
  Constant17/1 -> Multiport Switch4/4
  Constant18/1 -> Multiport Switch4/5
  Constant21/1 -> GetBit/1
  GetBit/1 -> Switch2/2, Switch1/2, Switch/2
  Multiport Switch/1 -> Product/2, Switch/3
  Multiport Switch1/1 -> Product1/2, Switch1/3
  WESDem_KpCorFac_mp/1 -> Product2/1, Product1/1, Product/1
  Product/1 -> Switch/1
  Product1/1 -> Switch1/1
  Multiport Switch2/1 -> Product2/2, Switch2/3
  Product2/1 -> Switch2/1
  Switch/1 -> Signal Conversion/1, WESDem_KpCurrHi_mp/1
  Switch1/1 -> WESDem_KpPosCurrHi_mp/1, Signal Conversion1/1
  Switch2/1 -> Signal Conversion2/1, WESDem_KpNegCurrHi_mp/1
  Multiport Switch3/1 -> Signal Conversion3/1, WESDem_PWinPosHi/1
  Multiport Switch4/1 -> Signal Conversion4/1, WESDem_PWinNegHi/1
  Signal Conversion/1 -> WESDem_KpCurrLo_mp/1
  Signal Conversion1/1 -> WESDem_KpPosCurrLo_mp/1
  Signal Conversion2/1 -> WESDem_KpNegCurrLo_mp/1
  Signal Conversion3/1 -> WESDem_PWinPosLo/1
  Signal Conversion4/1 -> WESDem_PWinNegLo/1

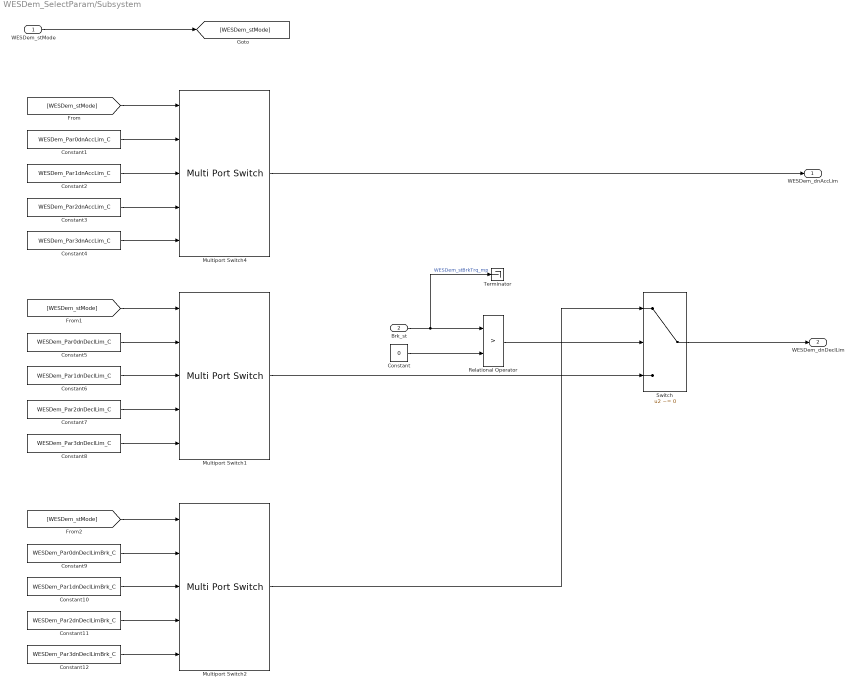
== system WESDem_SelectParam/Subsystem ==
  WESDem_stMode : Inport  Description=Operating mode of the working engine speed demand  OutMin=0  OutMax=255  OutDataTypeStr=State_uint8
  Brk_st : Inport  Description=Brake switch state  Port=2  OutMin=0  OutMax=255  OutDataTypeStr=State_uint8
  Constant : Constant  Value=0  OutDataTypeStr=Inherit: Inherit via back propagation
  Constant1 : Constant  Value=WESDem_Par0dnAccLim_C
  Constant10 : Constant  Value=WESDem_Par1dnDeclLimBrk_C
  Constant11 : Constant  Value=WESDem_Par2dnDeclLimBrk_C
  Constant12 : Constant  Value=WESDem_Par3dnDeclLimBrk_C
  Constant2 : Constant  Value=WESDem_Par1dnAccLim_C
  Constant3 : Constant  Value=WESDem_Par2dnAccLim_C
  Constant4 : Constant  Value=WESDem_Par3dnAccLim_C
  Constant5 : Constant  Value=WESDem_Par0dnDeclLim_C
  Constant6 : Constant  Value=WESDem_Par1dnDeclLim_C
  Constant7 : Constant  Value=WESDem_Par2dnDeclLim_C
  Constant8 : Constant  Value=WESDem_Par3dnDeclLim_C
  Constant9 : Constant  Value=WESDem_Par0dnDeclLimBrk_C
  Multiport Switch1 : MultiPortSwitch  DataPortOrder=Zero-based contiguous  Inputs=4
  Multiport Switch2 : MultiPortSwitch  DataPortOrder=Zero-based contiguous  Inputs=4
  Multiport Switch4 : MultiPortSwitch  DataPortOrder=Zero-based contiguous  Inputs=4
  Relational Operator : RelationalOperator  Operator=>  OutDataTypeStr=boolean  RndMeth=Simplest
  Switch : Switch  Criteria=u2 ~= 0
  Terminator : Terminator
  WESDem_dnAccLim : Outport  Tag=rpm/s  Description=Maximum permissible acceleration (Engine speed)  OutMin=-12000  OutMax=12000  OutDataTypeStr=EngSpeed_rpm_s
  WESDem_dnDeclLim : Outport  Tag=rpm/s  Description=Maximum permissible deceleration (Engine speed)  Port=2  OutMin=-12000  OutMax=12000  OutDataTypeStr=EngSpeed_rpm_s
  wires:
  WESDem_stMode/1 -> [WESDem_stMode]
  [WESDem_stMode] -> Multiport Switch4/1
  Constant1/1 -> Multiport Switch4/2
  Constant2/1 -> Multiport Switch4/3
  Constant3/1 -> Multiport Switch4/4
  Constant4/1 -> Multiport Switch4/5
  [WESDem_stMode] -> Multiport Switch1/1
  Constant5/1 -> Multiport Switch1/2
  Constant6/1 -> Multiport Switch1/3
  Constant7/1 -> Multiport Switch1/4
  Constant8/1 -> Multiport Switch1/5
  [WESDem_stMode] -> Multiport Switch2/1
  Constant9/1 -> Multiport Switch2/2
  Constant10/1 -> Multiport Switch2/3
  Constant11/1 -> Multiport Switch2/4
  Constant12/1 -> Multiport Switch2/5
  Brk_st/1 -> Terminator/1, Relational Operator/1  "WESDem_stBrkTrq_mp"
  Constant/1 -> Relational Operator/2
  Relational Operator/1 -> Switch/2
  Multiport Switch1/1 -> Switch/3
  Multiport Switch2/1 -> Switch/1
  Switch/1 -> WESDem_dnDeclLim/1
  Multiport Switch4/1 -> WESDem_dnAccLim/1

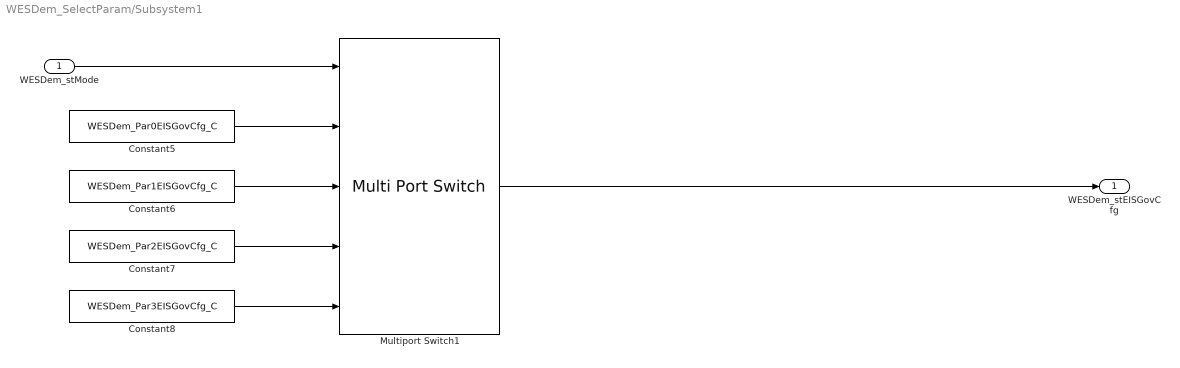
== system WESDem_SelectParam/Subsystem1 ==
  WESDem_stMode : Inport  Description=Operating mode of the working engine speed demand  OutMin=0  OutMax=255  OutDataTypeStr=State_uint8
  Constant5 : Constant  Value=WESDem_Par0EISGovCfg_C
  Constant6 : Constant  Value=WESDem_Par1EISGovCfg_C
  Constant7 : Constant  Value=WESDem_Par2EISGovCfg_C
  Constant8 : Constant  Value=WESDem_Par3EISGovCfg_C
  Multiport Switch1 : MultiPortSwitch  DataPortOrder=Zero-based contiguous  Inputs=4
  WESDem_stEISGovCfg : Outport  Description=Configuration of the EISGov  OutMin=0  OutMax=255  OutDataTypeStr=State_uint8
  wires:
  WESDem_stMode/1 -> Multiport Switch1/1
  Constant5/1 -> Multiport Switch1/2
  Constant6/1 -> Multiport Switch1/3
  Constant7/1 -> Multiport Switch1/4
  Constant8/1 -> Multiport Switch1/5
  Multiport Switch1/1 -> WESDem_stEISGovCfg/1

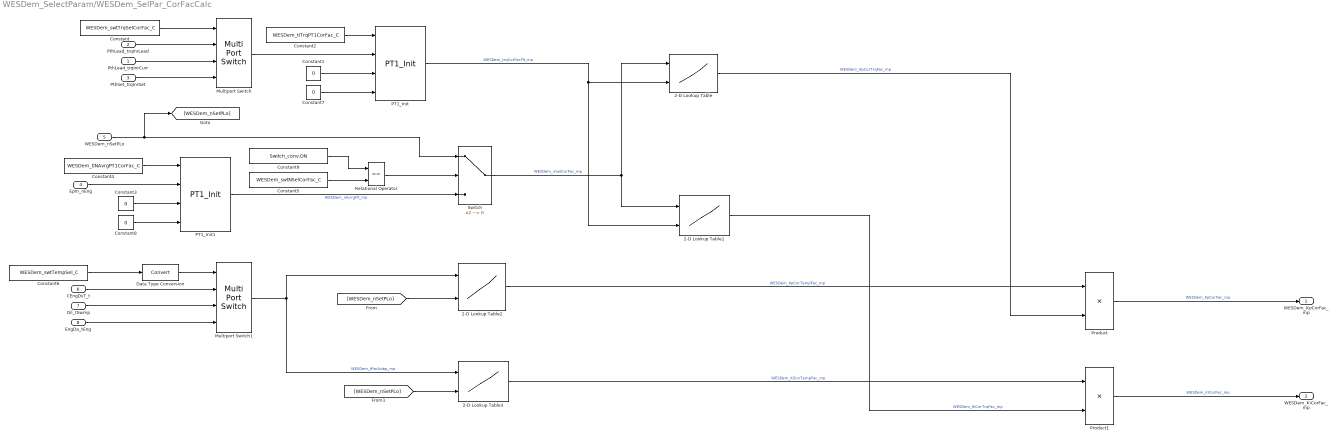
== system WESDem_SelectParam/WESDem_SelPar_CorFacCalc ==
  PthLead_trqInrCurr : Inport  Tag=Nm  Description=Actual percent engine torque  OutMin=-3000  OutMax=3000  OutDataTypeStr=Trq_Nm
  PthLead_trqInrLead : Inport  Tag=Nm  Description=Inner torque lead value  Port=2  OutMin=-3000  OutMax=3000  OutDataTypeStr=Trq_Nm
  PthSet_trqInrSet : Inport  Tag=Nm  Description=Inner torque set value after monitoring limitation  Port=3  OutMin=-3000  OutMax=3276.7  OutDataTypeStr=Trq_Nm
  Epm_nEng : Inport  Tag=rpm  Description=Engine speed  Port=4  OutMin=0  OutMax=6000  OutDataTypeStr=EngSpeed_rpm
  WESDem_nSetPLo : Inport  Tag=rpm  Description=Lower setpoint speed interval of WESDem  Port=5  OutMin=0  OutMax=6000  OutDataTypeStr=EngSpeed_rpm
  CEngDsT_t : Inport  Tag=deg  Description=engine coolant temperature after filter  Port=6  OutMin=-200  OutMax=200  OutDataTypeStr=Temp_deg
  Oil_tSwmp : Inport  Tag=deg  Description=Oil temperature in oil sump  Port=7  OutMin=-50  OutMax=200  OutDataTypeStr=Temp_deg
  EngDa_tEng : Inport  Tag=deg  Description=Engine temperature  Port=8  OutMin=-1000  OutMax=1000  OutDataTypeStr=Temp_deg
  2-D Lookup Table : Lookup_n-D  BreakpointsForDimension1=WESDem_KpCorTrqFac_MAPY  BreakpointsForDimension2=WESDem_KpCorTrqFac_MAPX  BeginIndexSearchUsingPreviousIndexResult=on  Table=WESDem_KpCorTrqFac_MAP  ExtrapMethod=Clip  UseLastTableValue=on  InternalRulePriority=Speed  OutDataTypeStr=Inherit: Inherit via back propagation  RndMeth=Simplest
  2-D Lookup Table1 : Lookup_n-D  BreakpointsForDimension1=WESDem_KiCorTrqFac_MAPY  BreakpointsForDimension2=WESDem_KiCorTrqFac_MAPX  BeginIndexSearchUsingPreviousIndexResult=on  Table=WESDem_KiCorTrqFac_MAP  ExtrapMethod=Clip  UseLastTableValue=on  InternalRulePriority=Speed  OutDataTypeStr=Inherit: Inherit via back propagation  RndMeth=Simplest  SaturateOnIntegerOverflow=on
  2-D Lookup Table2 : Lookup_n-D  BreakpointsForDimension1=WESDem_KpCorTempFac_MAPY  BreakpointsForDimension2=WESDem_KpCorTempFac_MAPX  BeginIndexSearchUsingPreviousIndexResult=on  Table=WESDem_KpCorTempFac_MAP  ExtrapMethod=Clip  UseLastTableValue=on  InternalRulePriority=Speed  OutDataTypeStr=Inherit: Inherit via back propagation  RndMeth=Simplest
  2-D Lookup Table3 : Lookup_n-D  BreakpointsForDimension1=WESDem_KiCorTempFac_MAPY  BreakpointsForDimension2=WESDem_KiCorTempFac_MAPX  BreakpointsForDimension2DataTypeStr=Inherit: Inherit from 'Breakpoint data'  BeginIndexSearchUsingPreviousIndexResult=on  Table=WESDem_KiCorTempFac_MAP  ExtrapMethod=Clip  UseLastTableValue=on  InternalRulePriority=Speed  OutDataTypeStr=Inherit: Inherit via back propagation  RndMeth=Simplest
  Constant : Constant  Value=WESDem_swtTrqSelCorFac_C
  Constant{1,3,7..8} (4 alike) : Constant  Value=0  OutDataTypeStr=Inherit: Inherit via back propagation
  Constant2 : Constant  Value=WESDem_tiTrqPT1CorFac_C
  Constant4 : Constant  Value=WESDem_tiNAvrgPT1CorFac_C
  Constant5 : Constant  Value=WESDem_swtNSelCorFac_C
  Constant6 : Constant  Value=WESDem_swtTempSel_C
  Constant9 : Constant  Value=Switch_conv.ON
  Data Type Conversion : DataTypeConversion
  Multiport Switch : MultiPortSwitch  DataPortOrder=Zero-based contiguous
  Multiport Switch1 : MultiPortSwitch  DataPortOrder=Zero-based contiguous
  PT1_Init : CXLib/PT1_Init
  PT1_Init1 : CXLib/PT1_Init
  Product : Product  OutDataTypeStr=Inherit: Inherit via back propagation  SaturateOnIntegerOverflow=on
  Product1 : Product  OutDataTypeStr=Inherit: Inherit via back propagation  SaturateOnIntegerOverflow=on
  Relational Operator : RelationalOperator  Operator===  OutDataTypeStr=boolean  RndMeth=Simplest
  Switch : Switch  Criteria=u2 ~= 0  OutDataTypeStr=Inherit: Inherit via back propagation
  WESDem_KpCorFac_mp : Outport
  WESDem_KiCorFac_mp : Outport  Port=2
  wires:
  PthLead_trqInrLead/1 -> Multiport Switch/2
  PthLead_trqInrCurr/1 -> Multiport Switch/3
  PthSet_trqInrSet/1 -> Multiport Switch/4
  Constant/1 -> Multiport Switch/1
  Multiport Switch/1 -> PT1_Init/2
  Constant1/1 -> PT1_Init/3
  Constant2/1 -> PT1_Init/1
  PT1_Init/1 -> 2-D Lookup Table/2, 2-D Lookup Table1/2  "WESDem_trqCorFacFlt_mp"
  Epm_nEng/1 -> PT1_Init1/2
  Constant3/1 -> PT1_Init1/3
  Constant4/1 -> PT1_Init1/1
  PT1_Init1/1 -> Switch/3  "WESDem_nAvrgFlt_mp"
  WESDem_nSetPLo/1 -> [WESDem_nSetPLo], Switch/1
  Switch/1 -> 2-D Lookup Table1/1, 2-D Lookup Table/1  "WESDem_nSelCorFac_mp"
  2-D Lookup Table/1 -> Product/2  "WESDem_KpCorTrqFac_mp"
  2-D Lookup Table1/1 -> Product1/2  "WESDem_KiCorTrqFac_mp"
  CEngDsT_t/1 -> Multiport Switch1/2
  Oil_tSwmp/1 -> Multiport Switch1/3
  EngDa_tEng/1 -> Multiport Switch1/4
  Constant6/1 -> Data Type Conversion/1
  Multiport Switch1/1 -> 2-D Lookup Table3/1, 2-D Lookup Table2/1  "WESDem_tParAdap_mp"
  [WESDem_nSetPLo] -> 2-D Lookup Table2/2
  2-D Lookup Table2/1 -> Product/1  "WESDem_KpCorTempFac_mp"
  [WESDem_nSetPLo] -> 2-D Lookup Table3/2
  2-D Lookup Table3/1 -> Product1/1  "WESDem_KiCorTempFac_mp"
  Product/1 -> WESDem_KpCorFac_mp/1  "WESDem_KpCorFac_mp"
  Product1/1 -> WESDem_KiCorFac_mp/1  "WESDem_KiCorFac_mp"
  Constant7/1 -> PT1_Init/4
  Constant8/1 -> PT1_Init1/4
  Data Type Conversion/1 -> Multiport Switch1/1
  Constant5/1 -> Relational Operator/2
  Constant9/1 -> Relational Operator/1
  Relational Operator/1 -> Switch/2

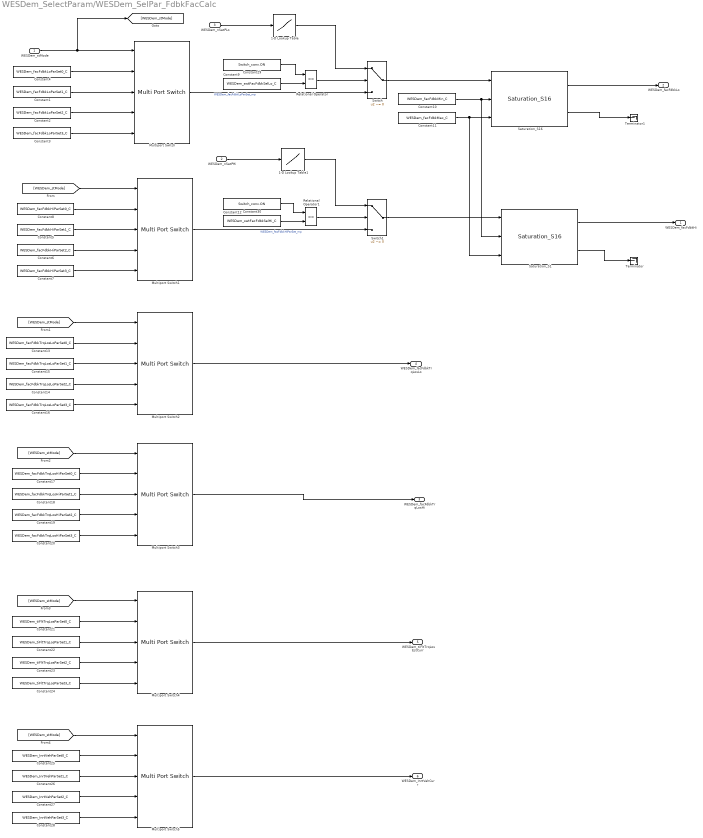
== system WESDem_SelectParam/WESDem_SelPar_FdbkFacCalc ==
  WESDem_stMode : Inport  Description=Operating mode of the working engine speed demand  OutMin=0  OutMax=255  OutDataTypeStr=State_uint8
  WESDem_nSetPHi : Inport  Tag=rpm  Description=Higher setpoint speed interval of WESDem  Port=2  OutMin=0  OutMax=6000  OutDataTypeStr=EngSpeed_rpm
  WESDem_nSetPLo : Inport  Tag=rpm  Description=Lower setpoint speed interval of WESDem  Port=3  OutMin=0  OutMax=6000  OutDataTypeStr=EngSpeed_rpm
  1-D Lookup Table : Lookup_n-D  NumberOfTableDimensions=1  BreakpointsForDimension1=WESDem_facFdbkLo_CURX  Table=WESDem_facFdbkLo_CUR  ExtrapMethod=Clip  InternalRulePriority=Speed  OutDataTypeStr=Inherit: Inherit via back propagation  RndMeth=Simplest
  1-D Lookup Table1 : Lookup_n-D  NumberOfTableDimensions=1  BreakpointsForDimension1=WESDem_facFdbkHi_CURX  Table=WESDem_facFdbkHi_CUR  ExtrapMethod=Clip  InternalRulePriority=Speed  OutDataTypeStr=Inherit: Inherit via back propagation  RndMeth=Simplest
  Constant1 : Constant  Value=WESDem_facFdbkLoParSet1_C
  Constant10 : Constant  Value=WESDem_facFdbkMin_C
  Constant11 : Constant  Value=WESDem_facFdbkMax_C
  Constant12 : Constant  Value=WESDem_swtFacFdbkSelHi_C
  Constant13 : Constant  Value=WESDem_facFdbkTrqLosLoParSet0_C
  Constant14 : Constant  Value=WESDem_facFdbkTrqLosLoParSet2_C
  Constant15 : Constant  Value=WESDem_facFdbkTrqLosLoParSet1_C
  Constant16 : Constant  Value=WESDem_facFdbkTrqLosLoParSet3_C
  Constant17 : Constant  Value=WESDem_facFdbkTrqLosHiParSet0_C
  Constant18 : Constant  Value=WESDem_facFdbkTrqLosHiParSet1_C
  Constant19 : Constant  Value=WESDem_facFdbkTrqLosHiParSet2_C
  Constant2 : Constant  Value=WESDem_facFdbkLoParSet2_C
  Constant20 : Constant  Value=WESDem_facFdbkTrqLosHiParSet3_C
  Constant21 : Constant  Value=WESDem_tiFltTrqLosParSet0_C
  Constant22 : Constant  Value=WESDem_tiFltTrqLosParSet1_C
  Constant23 : Constant  Value=WESDem_tiFltTrqLosParSet2_C
  Constant24 : Constant  Value=WESDem_tiFltTrqLosParSet3_C
  Constant25 : Constant  Value=WESDem_InrtVehParSet0_C
  Constant26 : Constant  Value=WESDem_InrtVehParSet1_C
  Constant27 : Constant  Value=WESDem_InrtVehParSet2_C
  Constant28 : Constant  Value=WESDem_InrtVehParSet3_C
  Constant29 : Constant  Value=Switch_conv.ON
  Constant3 : Constant  Value=WESDem_facFdbkLoParSet3_C
  Constant30 : Constant  Value=Switch_conv.ON
  Constant4 : Constant  Value=WESDem_facFdbkLoParSet0_C
  Constant5 : Constant  Value=WESDem_facFdbkHiParSet1_C
  Constant6 : Constant  Value=WESDem_facFdbkHiParSet2_C
  Constant7 : Constant  Value=WESDem_facFdbkHiParSet3_C
  Constant8 : Constant  Value=WESDem_facFdbkHiParSet0_C
  Constant9 : Constant  Value=WESDem_swtFacFdbkSelLo_C
  Multiport Switch{,1..5} (6 alike) : MultiPortSwitch  DataPortOrder=Zero-based contiguous  Inputs=4
  Relational Operator : RelationalOperator  Operator===  OutDataTypeStr=boolean  RndMeth=Simplest
  Relational Operator1 : RelationalOperator  Operator===  OutDataTypeStr=boolean  RndMeth=Simplest
  Saturation_S1 : CXLib/Saturation_S16
  Saturation_S16 : CXLib/Saturation_S16
  Switch : Switch  Criteria=u2 ~= 0
  Switch1 : Switch  Criteria=u2 ~= 0
  Terminator : Terminator
  Terminator1 : Terminator
  WESDem_facFdbkHi : Outport  Tag=rpm/Nm  Description=inner feedback factor for the upper setpoint  OutMin=-20  OutMax=20  OutDataTypeStr=FdbkNm2rpm_rpm_Nm
  WESDem_facFdbkLo : Outport  Tag=rpm/Nm  Description=inner feedback factor for the lower setpoint  Port=2  OutMin=-20  OutMax=20  OutDataTypeStr=FdbkNm2rpm_rpm_Nm
  WESDem_facFdbkTrqLosHi : Outport  Tag=rpm/Nm  Description=inner feedback factor for the upper setpoint  Port=3  OutMin=-20  OutMax=20  OutDataTypeStr=FdbkNm2rpm_rpm_Nm
  WESDem_facFdbkTrqLosLo : Outport  Tag=rpm/Nm  Description=inner feedback factor for the lower setpoint  Port=4  OutMin=-20  OutMax=20  OutDataTypeStr=FdbkNm2rpm_rpm_Nm
  WESDem_tiFltTrqLosEstCurr : Outport  Description=time constant (PT1-Filter) for EISGov torque loss estimation  Port=5  OutMin=0  OutMax=99.998  OutDataTypeStr=PT_fac
  WESDem_InrtVehCurr : Outport  Tag=Nm/(rpm/s)  Description=mass inertia for EISGov torque loss estimation  Port=6  OutMin=-50  OutMax=50  OutDataTypeStr=HLSDem_Inrt
  wires:
  WESDem_stMode/1 -> [WESDem_stMode], Multiport Switch/1
  Constant4/1 -> Multiport Switch/2
  Constant1/1 -> Multiport Switch/3
  Constant2/1 -> Multiport Switch/4
  Constant3/1 -> Multiport Switch/5
  Constant8/1 -> Multiport Switch1/2
  Constant5/1 -> Multiport Switch1/3
  Constant6/1 -> Multiport Switch1/4
  Constant7/1 -> Multiport Switch1/5
  Multiport Switch/1 -> Switch/3  "WESDem_facFdbkLoParSet_mp"
  Multiport Switch1/1 -> Switch1/3  "WESDem_facFdbkHiParSet_mp"
  WESDem_nSetPLo/1 -> 1-D Lookup Table/1
  1-D Lookup Table/1 -> Switch/1
  Switch/1 -> Saturation_S16/1
  Constant10/1 -> Saturation_S1/2, Saturation_S16/2
  Constant11/1 -> Saturation_S1/3, Saturation_S16/3
  Saturation_S16/1 -> WESDem_facFdbkLo/1
  WESDem_nSetPHi/1 -> 1-D Lookup Table1/1
  1-D Lookup Table1/1 -> Switch1/1
  Switch1/1 -> Saturation_S1/1
  Saturation_S1/1 -> WESDem_facFdbkHi/1
  Saturation_S1/2 -> Terminator/1
  Saturation_S16/2 -> Terminator1/1
  [WESDem_stMode] -> Multiport Switch1/1
  [WESDem_stMode] -> Multiport Switch2/1
  Constant13/1 -> Multiport Switch2/2
  Constant14/1 -> Multiport Switch2/4
  Constant15/1 -> Multiport Switch2/3
  Constant16/1 -> Multiport Switch2/5
  [WESDem_stMode] -> Multiport Switch3/1
  Constant17/1 -> Multiport Switch3/2
  Constant18/1 -> Multiport Switch3/3
  Constant19/1 -> Multiport Switch3/4
  Constant20/1 -> Multiport Switch3/5
  Multiport Switch2/1 -> WESDem_facFdbkTrqLosLo/1
  Multiport Switch3/1 -> WESDem_facFdbkTrqLosHi/1
  [WESDem_stMode] -> Multiport Switch4/1
  Constant21/1 -> Multiport Switch4/2
  Constant22/1 -> Multiport Switch4/3
  Constant23/1 -> Multiport Switch4/4
  Constant24/1 -> Multiport Switch4/5
  Multiport Switch4/1 -> WESDem_tiFltTrqLosEstCurr/1
  [WESDem_stMode] -> Multiport Switch5/1
  Constant25/1 -> Multiport Switch5/2
  Constant26/1 -> Multiport Switch5/3
  Constant27/1 -> Multiport Switch5/4
  Constant28/1 -> Multiport Switch5/5
  Multiport Switch5/1 -> WESDem_InrtVehCurr/1
  Relational Operator/1 -> Switch/2
  Constant9/1 -> Relational Operator/2
  Constant29/1 -> Relational Operator/1
  Relational Operator1/1 -> Switch1/2
  Constant12/1 -> Relational Operator1/2
  Constant30/1 -> Relational Operator1/1
